simulink model "satellite_adcs_model"  (R2014b)
settings: Solver=ode3  StartTime=0.0  StopTime=tdur  FixedStep=dt  RelTol=1e-3
values from neighbouring files (symbols this model uses):
  CTRL_DT_MODE = 3    [satellite_adcs_run.m]
  CTRL_PT1_MODE = 5    [satellite_adcs_run.m]
  CTRL_PT2_MODE = 5    [satellite_adcs_run.m]
  CTRL_SWITCH1 = 1    [satellite_adcs_run.m]
  CTRL_SWITCH2 = P/2    [satellite_adcs_run.m]
  dt = CONST.dt    [extended_kalman_filter.m]    (also in filter_kalman_extended.m; filter_kalman_sequential.m; filter_kalman_unscented.m; satellite_adcs_run.m = 1)
  dt_gyro = 0.1    [satellite_adcs_run.m]
  dt_mg = dt    (= 1)    [satellite_adcs_run.m]
  dt_ss = dt    (= 1)    [satellite_adcs_run.m]
  dt_st = dt    (= 1)    [satellite_adcs_run.m]
  dt_ts = dt    (= 1)    [satellite_adcs_run.m]
  GYRO_Bias = [0.5;0.2;-0.3]*pi/180    [satellite_adcs_run.m]
  q_B_I_0 = qinvert(q_I_B_0,'xyzw')    [satellite_adcs_run.m]
  R_G_B = dcm(2,pi/2)    [satellite_adcs_run.m]
  R_S1_B = dcm(SSaxis(1),SSangles(1))    [satellite_adcs_run.m]
  R_S2_B = dcm(SSaxis(2),SSangles(2))    [satellite_adcs_run.m]
  R_S3_B = dcm(SSaxis(3),SSangles(3))    [satellite_adcs_run.m]
  R_S4_B = dcm(SSaxis(4),SSangles(4))    [satellite_adcs_run.m]
  sigMag = 1.25e-7    (= 1.25e-07)    [satellite_adcs_run.m]
  sigSS = 0.01*pi/180    (= 0.000174532925199)    [satellite_adcs_run.m]
  Taero_toggle = 0    [satellite_adcs_run.m]
  Tcontrol_toggle = 1    [satellite_adcs_run.m]
  temp_coeff = [0.01; 0.02; 0.005]*pi/180    [satellite_adcs_run.m]
  temp_ref = 20    [satellite_adcs_run.m]
  Tgg_toggle = 0    [satellite_adcs_run.m]
  Tsolar_toggle = 0    [satellite_adcs_run.m]
  Ug = dcm(3,GYRO_Mis(3))*dcm(2,GYRO_Mis(2))*dcm(1,GYRO_Mis(1))    [satellite_adcs_run.m]
  Umg = eye(3) + Gmg    [satellite_adcs_run.m]    (also in sensor_mag.m = CONST.Umg)
  update_st1 = 2    [satellite_adcs_run.m]
  update_st2 = 2    [satellite_adcs_run.m]
  Var_ARW = N_ARW^2    (= 2.56183250041e-09)    [satellite_adcs_run.m]
  Var_RRW = K_RRW^2/3    (= 4.06156559716e-12)    [satellite_adcs_run.m]
  varTemp = sigTemp^2    (= 4e-06)    [satellite_adcs_run.m]
  VarW = N_W^2    (= 3.04617419787e-22)    [satellite_adcs_run.m]
  w_B_BI_0 = w_B_BO_0 + w_B_OI_0    [satellite_adcs_run.m]
  wdot_B_BI_tgt = [0;0;0]    [satellite_adcs_run.m]
undefined symbols (not defined in the file or in its folder): magnitude, R_0, V_0, varST_x, varST_y, varST_z
libraries: simulink x6
(part 1 of 2)
settings Model: Creator=Goh  LastModifiedBy=root
settings DataIOCC: LimitDataPoints=off  SaveTime=off
settings OptimizationCC: BlockReduction=off  BooleanDataType=off  UseDivisionForNetSlopeComputation=off  SimCompilerOptimization=off
settings DebuggingCC: SaveWithParameterizedLinksMsg=none  UnderspecifiedInitializationDetection=Classic  MergeDetectMultiDrivingBlocksExec=none  SignalResolutionControl=TryResolveAllWithWarning  SolverPrmCheckMsg=none  FcnCallInpInsideContextMsg=error  FrameProcessingCompatibilityMsg=error  SFExecutionAtInitializationDiag=none
settings HardwareCC: ProdBitPerSizeT=32  ProdBitPerPtrDiffT=32  TargetUnknown=on
settings RTWCC: RTWCompilerOptimization=off
settings CodeAppCC: StateflowObjectComments=on
settings ConfigComp: CovMetricSettings=dw  CovHtmlReporting=on  CovSaveCumulativeToWorkspaceVar=on  CovSaveSingleToWorkspaceVar=on  CovExternalEMLEnable=off  CovSFcnEnable=off

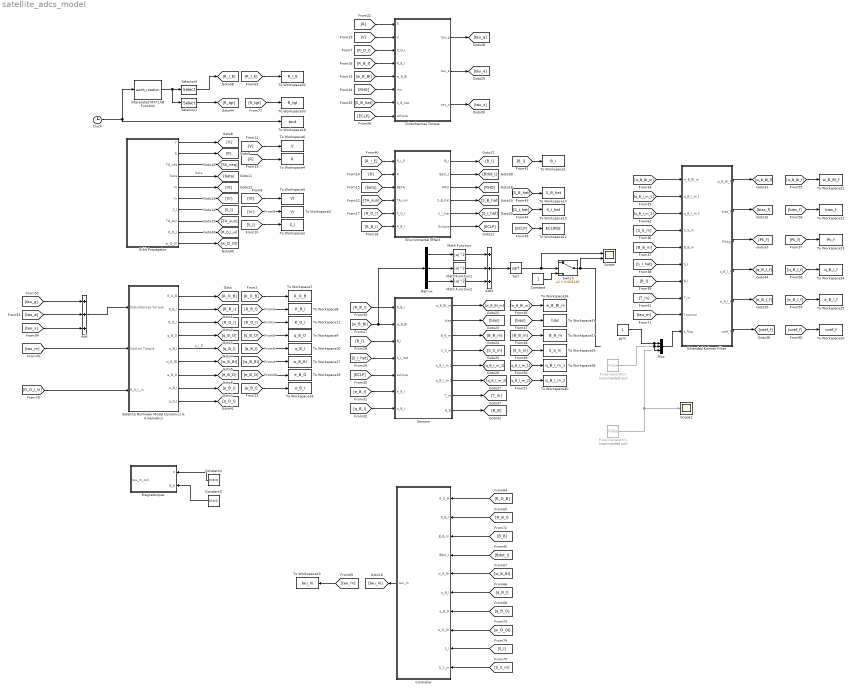
== system satellite_adcs_model ==
  Add : Sum  Inputs=+++
  Add1 : Sum  Inputs=3
  Clock : Clock
  Constant : Constant
  Constant3 : Constant  Value=[0;0;0]
  Constant4 : Constant  Value=[0;0;0]
  Controller : Subsystem
  Demux : Demux  Outputs=3
  Disturbances Torque : Subsystem
  Environmental Effect : Subsystem
  Extended Kalman Filter : Subsystem
  Interpreted MATLAB Function : MATLABFcn  MATLABFcn=earth_rotation  OutputDimensions=[3,4]  Output1D=off
  Magnetorquer : Subsystem
  Math Function : Math  Operator=magnitude^2  SaturateOnIntegerOverflow=on
  Math Function1 : Math  Operator=magnitude^2  SaturateOnIntegerOverflow=on
  Math Function2 : Math  Operator=magnitude^2  SaturateOnIntegerOverflow=on
  Mux : Mux  Inputs=3
  Orbit Propagator : Subsystem
  Pulse Generator : DiscretePulseGenerator  Commented=on  PulseType=Time based  Period=update_st1  PulseWidth=dt/update_st1*100
  Pulse Generator1 : DiscretePulseGenerator  Commented=on  PulseType=Time based  Period=update_st2  PulseWidth=dt/update_st2*100
  Satellite Nonlinear Model Dynamics & Kinematics : Subsystem
  Scope : Scope  NumInputPorts=2
  Scope1 : Scope
  Selector1 : Selector  NumberOfDimensions=2  InputPortWidth=9  IndexOptions=Index vector (dialog),Index vector (dialog)  Indices=1:3,4  OutputSizes=1,1
  Selector5 : Selector  NumberOfDimensions=2  InputPortWidth=9  IndexOptions=Index vector (dialog),Index vector (dialog)  Indices=1:3,1:3  OutputSizes=1,1
  Sensors : Subsystem
  Sqrt : Sqrt  SaturateOnIntegerOverflow=on
  Switch : Switch  Criteria=u2 > Threshold  Threshold=0.005236
  To Workspace1 : ToWorkspace  VariableName=B_I  SampleTime=dt
  To Workspace10 : ToWorkspace  VariableName=q_B_I  SampleTime=dt
  To Workspace11 : ToWorkspace  VariableName=R_O_I  SampleTime=dt
  To Workspace12 : ToWorkspace  VariableName=ECLIPSE  SampleTime=dt
      settings: Save2DSignal=2-D array (concatenate along first dimension)
  To Workspace13 : ToWorkspace  VariableName=S_I_hat  SampleTime=dt
  To Workspace14 : ToWorkspace  VariableName=S_B_hat  SampleTime=dt
  To Workspace15 : ToWorkspace  VariableName=tau_m  SampleTime=-1
  To Workspace16 : ToWorkspace  VariableName=tout  SampleTime=dt
  To Workspace17 : ToWorkspace  VariableName=w_B_BI  SampleTime=dt
  To Workspace18 : ToWorkspace  VariableName=e_B_I  SampleTime=dt
  To Workspace19 : ToWorkspace  VariableName=e_B_O  SampleTime=dt
  To Workspace2 : ToWorkspace  VariableName=S_I  SampleTime=dt
  To Workspace20 : ToWorkspace  VariableName=coef_f  SampleTime=dt
  To Workspace21 : ToWorkspace  VariableName=w_B_BI_f  SampleTime=dt
  To Workspace22 : ToWorkspace  VariableName=bias_f  SampleTime=dt
  To Workspace23 : ToWorkspace  VariableName=Pk_f  SampleTime=dt
  To Workspace24 : ToWorkspace  VariableName=q_B_I_f  SampleTime=dt
  To Workspace25 : ToWorkspace  VariableName=e_B_I_f  SampleTime=dt
  To Workspace26 : ToWorkspace  VariableName=w_B_BI_m  SampleTime=dt
  To Workspace27 : ToWorkspace  VariableName=B_B_m  SampleTime=dt
  To Workspace28 : ToWorkspace  VariableName=q_B_I_m_1  SampleTime=dt
  To Workspace29 : ToWorkspace  VariableName=S_S_m  SampleTime=dt
  To Workspace3 : ToWorkspace  VariableName=Vr  SampleTime=dt
  To Workspace30 : ToWorkspace  VariableName=q_B_I_m_2  SampleTime=dt
  To Workspace31 : ToWorkspace  VariableName=bias  SampleTime=dt
  To Workspace32 : ToWorkspace  VariableName=R_I_E  SampleTime=dt
  To Workspace33 : ToWorkspace  VariableName=R_tgt  SampleTime=dt
  To Workspace4 : ToWorkspace  VariableName=R  SampleTime=dt
  To Workspace5 : ToWorkspace  VariableName=Vt  SampleTime=dt
  To Workspace6 : ToWorkspace  VariableName=V  SampleTime=dt
  To Workspace7 : ToWorkspace  VariableName=R_O_B  SampleTime=dt
  To Workspace8 : ToWorkspace  VariableName=R_B_I  SampleTime=dt
  To Workspace9 : ToWorkspace  VariableName=q_B_O  SampleTime=dt
  "gyro " : Constant
  wires:
  Satellite Nonlinear Model Dynamics & Kinematics/1(R_O_B) -> [R_O_B]
  Satellite Nonlinear Model Dynamics & Kinematics/2(R_B_I) -> [R_B_I]
  Satellite Nonlinear Model Dynamics & Kinematics/4(q_B_O) -> [q_B_O]
  Satellite Nonlinear Model Dynamics & Kinematics/5(q_B_I) -> [q_B_I]  "q_I_B"
  Satellite Nonlinear Model Dynamics & Kinematics/6(w_B_BI) -> [w_B_BI]
  Satellite Nonlinear Model Dynamics & Kinematics/7(e_B_O) -> [e_B_O]
  Satellite Nonlinear Model Dynamics & Kinematics/8(e_B_I) -> [e_B_I]
  Orbit Propagator/7("S_I ") -> [S_I]
  Orbit Propagator/8(TA_sun) -> [TA_sun]
  Orbit Propagator/1(V) -> [V]
  Orbit Propagator/2(R) -> [R]
  Orbit Propagator/3(TA_veq) -> [TA_veq]
  Orbit Propagator/4(beta) -> [beta]  "beta"
  Orbit Propagator/5(Vt) -> [Vt]
  Orbit Propagator/6(Vr) -> [Vr]
  Environmental Effect/1(B_I) -> [B_I]
  Environmental Effect/3(RHO) -> [RHO]
  Environmental Effect/4(S_B_hat) -> [S_B_hat]
  Environmental Effect/5(S_I_hat) -> [S_I_hat]
  Environmental Effect/6(Eclipse) -> [ECLP]
  Sensors/3(B_B_m) -> [B_B_m]
  Sensors/2(bias) -> [bias]
  Sensors/1(w_B_BI_m) -> [w_B_BI_m]
  Sensors/4(S_S_m) -> [S_S_m]
  Sensors/5(q_B_I_m 1) -> [q_B_I_m_1]
  Disturbances Torque/1(tau_g) -> [tau_g]
  Disturbances Torque/2(tau_a) -> [tau_a]
  Disturbances Torque/3(tau_s) -> [tau_s]
  Extended Kalman Filter/1(w_B_BI_f) -> [w_B_BI_f]
  Extended Kalman Filter/2(bias_f) -> [bias_f]
  Extended Kalman Filter/3(Pdiag) -> [Pk_f]
  Extended Kalman Filter/4(q_B_I_f) -> [q_B_I_f]
  Extended Kalman Filter/5(e_B_I_f) -> [e_B_I_f]
  [R_O_B] -> To Workspace7/1
  [R_B_I] -> To Workspace8/1
  [R_O_I] -> To Workspace11/1
  [q_B_O] -> To Workspace9/1
  [q_B_I] -> To Workspace10/1
  [w_B_BI] -> To Workspace17/1
  [e_B_O] -> To Workspace19/1
  [e_B_I] -> To Workspace18/1
  [Vt] -> To Workspace5/1
  [Vr] -> To Workspace3/1
  [S_I] -> To Workspace2/1
  [R] -> To Workspace4/1
  [V] -> To Workspace6/1
  [beta] -> Environmental Effect/3(BETA)
  [TA_sun] -> Environmental Effect/4(TA_sun)
  [R] -> Environmental Effect/2(R)
  [R_O_I] -> Environmental Effect/5(R_O_I)
  [R_B_I] -> Environmental Effect/6(R_B_I)
  [RHO] -> Disturbances Torque/6(rho)
  [w_B_BI] -> Disturbances Torque/5(w_B_BI)
  [R_B_I] -> Disturbances Torque/4(R_B_I)
  [R_O_I] -> Disturbances Torque/3(R_O_I)
  [V] -> Disturbances Torque/2(V)
  [R] -> Disturbances Torque/1(R)
  [S_B_hat] -> Disturbances Torque/7(S_B_hat)
  [ECLP] -> Disturbances Torque/8(eclipse)
  [R_B_I] -> Sensors/1(R_B_I)
  [w_B_BI] -> Demux/1, Sensors/2(w_B_BI)
  [B_I] -> Sensors/3(B_I)
  [e_B_I] -> Sensors/6(e_B_I)
  [q_B_I] -> Sensors/7(q_B_I)
  [S_I_hat] -> Sensors/4(S_I_hat)
  [ECLP] -> Sensors/5(eclipse)
  [B_B_m] -> Extended Kalman Filter/5(B_B_m)
  [S_I_hat] -> Extended Kalman Filter/6(S_I)
  [B_I] -> Extended Kalman Filter/7(B_I)
  [S_S_m] -> Extended Kalman Filter/4(S_S_m)
  [w_B_BI_m] -> Extended Kalman Filter/1(w_B_BI_m)
  [q_B_I_m_1] -> Extended Kalman Filter/2(q_B_I_m 1)
  [B_I] -> To Workspace1/1
  [S_B_hat] -> To Workspace14/1
  [S_I_hat] -> To Workspace13/1
  [ECLP] -> To Workspace12/1
  [w_B_BI_m] -> To Workspace26/1
  [q_B_I_m_1] -> To Workspace28/1
  [bias] -> To Workspace31/1
  [S_S_m] -> To Workspace29/1
  [B_B_m] -> To Workspace27/1
  [tau_s] -> Add/3
  [tau_g] -> Add/1
  [w_B_BI_f] -> To Workspace21/1
  [bias_f] -> To Workspace22/1
  [Pk_f] -> To Workspace23/1
  [q_B_I_f] -> To Workspace24/1
  [e_B_I_f] -> To Workspace25/1
  [coef_f] -> To Workspace20/1
  Extended Kalman Filter/6(coef_f) -> [coef_f]
  Sensors/7(T_m) -> [T_m]
  [T_m] -> Extended Kalman Filter/8(T_m)
  [q_B_I_m_2] -> To Workspace30/1
  Sensors/6(q_B_I_m 2) -> [q_B_I_m_2]
  [q_B_I_m_2] -> Extended Kalman Filter/3(q_B_I_m 2)
  [tau_a] -> Add/2
  [R_I_E] -> To Workspace32/1
  [R_I_E] -> Environmental Effect/1(R_I_E)
  Mux/1 -> Extended Kalman Filter/10(s_flag)
  [w_B_BI] -> Controller/5(w_B_BI)
  [tau_m] -> To Workspace15/1
  Controller/1(tau_m) -> [tau_m]
  [R_O_B] -> Controller/1(R_O_B)
  [B_B] -> Controller/3(B_B_m)
  [R_B_I] -> Controller/2(R_B_I)
  [tau_m] -> Extended Kalman Filter/9(Tcontrol)
  Environmental Effect/2(Bdot_I) -> [Bdot_I]
  [Bdot_I] -> Controller/4(Bdot_I)
  "gyro "/1 -> Mux/3, Mux/2, Mux/1
  Pulse Generator1/1 -> Scope1/1
  Switch/1 -> Scope/2
  Demux/1 -> Math Function/1
  Demux/2 -> Math Function1/1
  Demux/3 -> Math Function2/1
  Math Function/1 -> Add1/1
  Math Function1/1 -> Add1/2
  Math Function2/1 -> Add1/3
  Add1/1 -> Sqrt/1
  Sqrt/1 -> Switch/2, Scope/1
  Constant/1 -> Switch/3
  Clock/1 -> To Workspace16/1, Interpreted MATLAB Function/1
  [q_B_I] -> Controller/6(q_B_I)
  [q_B_O] -> Controller/7(q_B_O)
  Satellite Nonlinear Model Dynamics & Kinematics/9(q_O_I) -> [q_O_I]
  Satellite Nonlinear Model Dynamics & Kinematics/3(R_O_I) -> [R_O_I]
  Orbit Propagator/10(w_O_OI) -> [w_O_OI]
  [w_O_OI] -> Controller/8(w_O_OI)
  [S_I] -> Controller/9(S_I)
  [S_S_m] -> Controller/10(S_S_m)
  Pulse Generator/1 -> ?
  Constant4/1 -> Magnetorquer/1(V)
  Constant3/1 -> Magnetorquer/2(B_b)
  Sensors/8(B_B) -> [B_B]
  Orbit Propagator/9(R_O_I) -> [R_O_I_in]
  [R_O_I_in] -> Satellite Nonlinear Model Dynamics & Kinematics/3(R_O_I_in)
  Add/1 -> Satellite Nonlinear Model Dynamics & Kinematics/1(Disturbances Torque)
  Interpreted MATLAB Function/1 -> Selector1/1, Selector5/1
  [tau_m] -> Satellite Nonlinear Model Dynamics & Kinematics/2(Control Torque)
  [R_tgt] -> To Workspace33/1
  Selector5/1 -> [R_I_E]
  Selector1/1 -> [R_tgt]

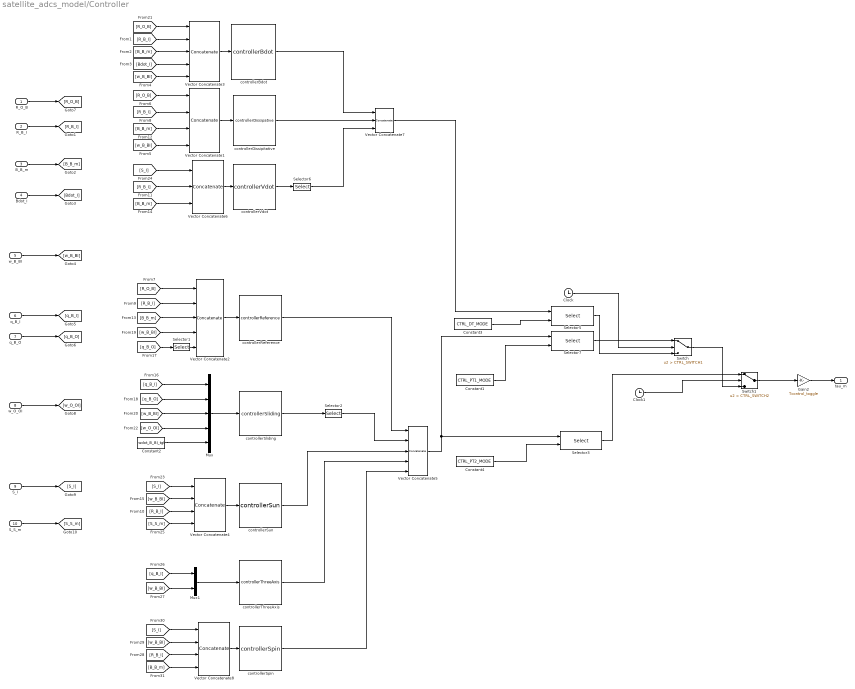
== system satellite_adcs_model/Controller ==
  R_O_B : Inport
  R_B_I : Inport  Port=2
  B_B_m : Inport  Port=3
  Bdot_I : Inport  Port=4
  w_B_BI : Inport  Port=5
  q_B_I : Inport  Port=6
  q_B_O : Inport  Port=7
  w_O_OI : Inport  Port=8
  S_I : Inport  Port=9
  S_S_m : Inport  Port=10
  Clock : Clock
  Clock1 : Clock
  Constant1 : Constant  Value=CTRL_PT1_MODE  VectorParams1D=off
  Constant2 : Constant  Value=wdot_B_BI_tgt  VectorParams1D=off
  Constant3 : Constant  Value=CTRL_DT_MODE  VectorParams1D=off
  Constant4 : Constant  Value=CTRL_PT2_MODE  VectorParams1D=off
  Gain2 : Gain  Gain=Tcontrol_toggle
  Mux : Mux  Inputs=5
  Mux1 : Mux  Inputs=2
  Selector1 : Selector  NumberOfDimensions=2  InputPortWidth=3  IndexOptions=Index vector (dialog),Index vector (dialog)  Indices=[1:3],1  OutputSizes=1,1
  Selector2 : Selector  NumberOfDimensions=2  InputPortWidth=3  IndexOptions=Index vector (dialog),Index vector (dialog)  Indices=[1:3],1  OutputSizes=1,1
  Selector3 : Selector  NumberOfDimensions=2  InputPortWidth=3  IndexOptions=Select all,Index vector (port)  Indices=[1 3],1  OutputSizes=1,1
  Selector5 : Selector  NumberOfDimensions=2  InputPortWidth=3  IndexOptions=Select all,Index vector (port)  Indices=[1 3],1  OutputSizes=1,1
  Selector6 : Selector  NumberOfDimensions=2  InputPortWidth=3  IndexOptions=Index vector (dialog),Index vector (dialog)  Indices=[1:3],1  OutputSizes=1,1
  Selector7 : Selector  NumberOfDimensions=2  InputPortWidth=3  IndexOptions=Select all,Index vector (port)  Indices=[1 3],1  OutputSizes=1,1
  Switch : Switch  Criteria=u2 > Threshold  Threshold=CTRL_SWITCH1
  Switch1 : Switch  Criteria=u2 > Threshold  Threshold=CTRL_SWITCH2
  Vector Concatenate1 : Concatenate  NumInputs=4  Mode=Multidimensional array  ConcatenateDimension=2
  Vector Concatenate2 : Concatenate  NumInputs=5  Mode=Multidimensional array  ConcatenateDimension=2
  Vector Concatenate3 : Concatenate  NumInputs=5  Mode=Multidimensional array  ConcatenateDimension=2
  Vector Concatenate4 : Concatenate  NumInputs=4  Mode=Multidimensional array  ConcatenateDimension=2
  Vector Concatenate5 : Concatenate  NumInputs=5  Mode=Multidimensional array  ConcatenateDimension=2
  Vector Concatenate6 : Concatenate  NumInputs=3  Mode=Multidimensional array  ConcatenateDimension=2
  Vector Concatenate7 : Concatenate  NumInputs=3  Mode=Multidimensional array  ConcatenateDimension=2
  Vector Concatenate8 : Concatenate  NumInputs=4  Mode=Multidimensional array  ConcatenateDimension=2
  controllerBdot : MATLABFcn  MATLABFcn=controllerBdot  OutputDimensions=[3,1]  Output1D=off
  controllerDissipitative : MATLABFcn  MATLABFcn=controllerDissipative  OutputDimensions=[3,1]  Output1D=off
  controllerReference : MATLABFcn  MATLABFcn=controllerReference  OutputDimensions=[3,1]  Output1D=off
  "controllerSliding " : MATLABFcn  MATLABFcn=controllerSliding  OutputDimensions=[3,3]  Output1D=off
  controllerSpin : MATLABFcn  MATLABFcn=controllerSpin  OutputDimensions=[3,1]  Output1D=off
  controllerSun : MATLABFcn  MATLABFcn=controllerSun  OutputDimensions=[3,1]  Output1D=off
  controllerThreeAxis : MATLABFcn  MATLABFcn=controllerThreeAxis  OutputDimensions=[3,1]  Output1D=off
  controllerVdot : MATLABFcn  MATLABFcn=controllerVdot  OutputDimensions=[6,1]  Output1D=off
  tau_m : Outport
  wires:
  Vector Concatenate1/1 -> controllerDissipitative/1
  R_O_B/1 -> [R_O_B]
  R_B_I/1 -> [R_B_I]
  B_B_m/1 -> [B_B_m]
  w_B_BI/1 -> [w_B_BI]
  Vector Concatenate2/1 -> controllerReference/1
  controllerReference/1 -> Vector Concatenate5/1
  Clock/1 -> Switch/2
  Switch/1 -> Switch1/3
  Vector Concatenate3/1 -> controllerBdot/1
  controllerBdot/1 -> Vector Concatenate7/1
  controllerDissipitative/1 -> Vector Concatenate7/2
  Vector Concatenate7/1 -> Selector5/1
  Mux/1 -> "controllerSliding "/1
  Constant2/1 -> Mux/5
  Selector7/1 -> Switch/1
  Vector Concatenate4/1 -> controllerSun/1
  Vector Concatenate5/1 -> Selector3/1, Selector7/1
  Selector1/1 -> Vector Concatenate2/5
  "controllerSliding "/1 -> Selector2/1
  Selector2/1 -> Vector Concatenate5/2
  controllerSun/1 -> Vector Concatenate5/3
  Constant1/1 -> Selector7/2
  Vector Concatenate6/1 -> controllerVdot/1
  controllerVdot/1 -> Selector6/1
  Selector5/1 -> Switch/3
  Constant3/1 -> Selector5/2
  Selector6/1 -> Vector Concatenate7/3
  [R_O_B] -> Vector Concatenate3/1
  [R_B_I] -> Vector Concatenate3/2
  [B_B_m] -> Vector Concatenate3/3
  [Bdot_I] -> Vector Concatenate3/4
  Bdot_I/1 -> [Bdot_I]
  [w_B_BI] -> Vector Concatenate3/5
  [w_B_BI] -> Vector Concatenate1/4
  [R_O_B] -> Vector Concatenate1/1
  [R_O_B] -> Vector Concatenate2/1
  [R_B_I] -> Vector Concatenate1/2
  [R_B_I] -> Vector Concatenate2/2
  [R_B_I] -> Vector Concatenate4/3
  [R_B_I] -> Vector Concatenate6/2
  [B_B_m] -> Vector Concatenate1/3
  [B_B_m] -> Vector Concatenate2/3
  [B_B_m] -> Vector Concatenate6/3
  [w_B_BI] -> Vector Concatenate4/2
  q_B_I/1 -> [q_B_I]
  [q_B_I] -> Mux/1
  q_B_O/1 -> [q_B_O]
  [q_B_O] -> Selector1/1
  [q_B_O] -> Mux/2
  [w_B_BI] -> Vector Concatenate2/4
  [w_B_BI] -> Mux/3
  w_O_OI/1 -> [w_O_OI]
  [w_O_OI] -> Mux/4
  S_I/1 -> [S_I]
  [S_I] -> Vector Concatenate4/1
  [S_I] -> Vector Concatenate6/1
  S_S_m/1 -> [S_S_m]
  [S_S_m] -> Vector Concatenate4/4
  controllerThreeAxis/1 -> Vector Concatenate5/4
  Mux1/1 -> controllerThreeAxis/1
  [q_B_I] -> Mux1/1
  [w_B_BI] -> Mux1/2
  Clock1/1 -> Switch1/2
  Switch1/1 -> Gain2/1
  Selector3/1 -> Switch1/1
  Constant4/1 -> Selector3/2
  Gain2/1 -> tau_m/1
  Vector Concatenate8/1 -> controllerSpin/1
  [w_B_BI] -> Vector Concatenate8/2
  [S_I] -> Vector Concatenate8/1
  [R_B_I] -> Vector Concatenate8/3
  [B_B_m] -> Vector Concatenate8/4
  controllerSpin/1 -> Vector Concatenate5/5

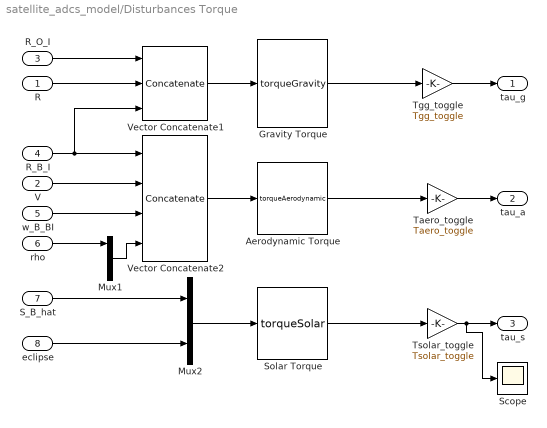
== system satellite_adcs_model/Disturbances Torque ==
  R : Inport
  V : Inport  Port=2
  R_O_I : Inport  Port=3
  R_B_I : Inport  Port=4
  w_B_BI : Inport  Port=5
  rho : Inport  Port=6
  S_B_hat : Inport  Port=7
  eclipse : Inport  Port=8
  Aerodynamic Torque : MATLABFcn  MATLABFcn=torqueAerodynamic  OutputDimensions=[3,1]  Output1D=off
  Gravity Torque : MATLABFcn  MATLABFcn=torqueGravity  OutputDimensions=[3,1]  Output1D=off
  Mux1 : Mux  Inputs=3
  Mux2 : Mux  Inputs=2
  Scope : Scope
      settings: YMin=-0.0000000000000000000000009  YMax=0.0000000000000000000000012  SaveName=ScopeData8
  Solar Torque : MATLABFcn  MATLABFcn=torqueSolar  OutputDimensions=[3,1]  Output1D=off
  Taero_toggle : Gain  Gain=Taero_toggle
  Tgg_toggle : Gain  Gain=Tgg_toggle
  Tsolar_toggle : Gain  Gain=Tsolar_toggle
  Vector Concatenate1 : Concatenate  NumInputs=3  Mode=Multidimensional array  ConcatenateDimension=2
  Vector Concatenate2 : Concatenate  NumInputs=4  Mode=Multidimensional array  ConcatenateDimension=2
  tau_g : Outport
  tau_a : Outport  Port=2
  tau_s : Outport  Port=3
  wires:
  Vector Concatenate2/1 -> Aerodynamic Torque/1
  Mux1/1 -> Vector Concatenate2/4
  Solar Torque/1 -> Tsolar_toggle/1
  Vector Concatenate1/1 -> Gravity Torque/1
  Mux2/1 -> Solar Torque/1
  S_B_hat/1 -> Mux2/1
  w_B_BI/1 -> Vector Concatenate2/3
  R_B_I/1 -> Vector Concatenate1/3, Vector Concatenate2/1
  V/1 -> Vector Concatenate2/2
  R/1 -> Vector Concatenate1/2
  R_O_I/1 -> Vector Concatenate1/1
  rho/1 -> Mux1/1
  Aerodynamic Torque/1 -> Taero_toggle/1
  eclipse/1 -> Mux2/2
  Tgg_toggle/1 -> tau_g/1
  Taero_toggle/1 -> tau_a/1
  Tsolar_toggle/1 -> Scope/1, tau_s/1
  Gravity Torque/1 -> Tgg_toggle/1

== system satellite_adcs_model/Environmental Effect ==
  R_I_E : Inport
  R : Inport  Port=2
  BETA : Inport  Port=3
  TA_sun : Inport  Port=4
  R_O_I : Inport  Port=5
  R_B_I : Inport  Port=6
  DENSITY : Subsystem
  MAGNETIC FIELD : Subsystem
  SUN : Subsystem
  B_I : Outport
  Bdot_I : Outport  Port=2
  RHO : Outport  Port=3
  S_B_hat : Outport  Port=4
  S_I_hat : Outport  Port=5
  Eclipse : Outport  Port=6
  wires:
  R/1 -> MAGNETIC FIELD/2(R), SUN/1(R), DENSITY/1(R)
  TA_sun/1 -> SUN/2(S_TA), DENSITY/2(S_TA)
  BETA/1 -> SUN/3(BETA), DENSITY/3(BETA)
  R_O_I/1 -> SUN/4(R_O_I)
  R_B_I/1 -> SUN/5(R_B_I)
  SUN/1(S_B_hat) -> S_B_hat/1
  SUN/2(S_I_hat) -> S_I_hat/1
  SUN/3(Eclipse) -> Eclipse/1
  DENSITY/1(RHO) -> RHO/1
  R_I_E/1 -> MAGNETIC FIELD/1(R_I_E)
  MAGNETIC FIELD/1(B_I) -> B_I/1
  MAGNETIC FIELD/2(Bdot_I) -> Bdot_I/1

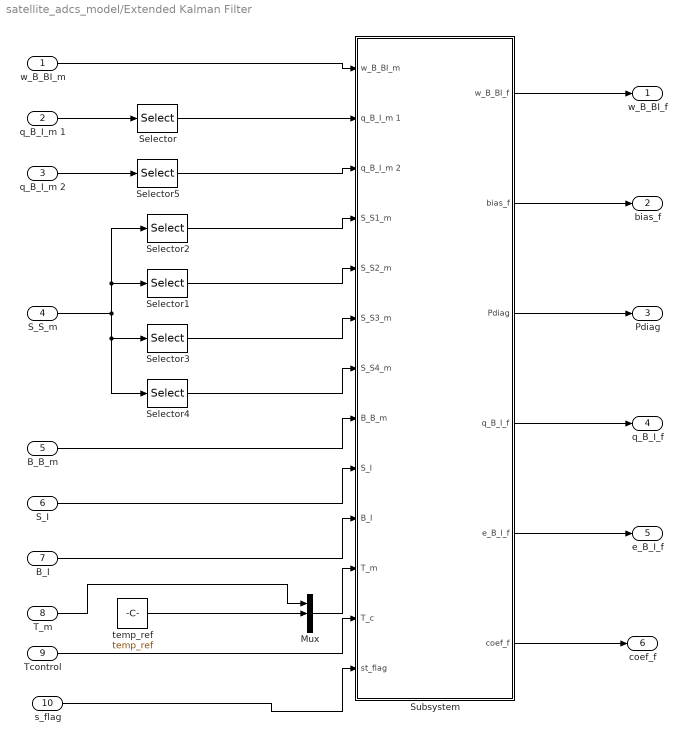
== system satellite_adcs_model/Extended Kalman Filter ==
  w_B_BI_m : Inport
  q_B_I_m 1 : Inport  Port=2
  q_B_I_m 2 : Inport  Port=3
  S_S_m : Inport  Port=4
  B_B_m : Inport  Port=5
  S_I : Inport  Port=6
  B_I : Inport  Port=7
  T_m : Inport  Port=8
  Tcontrol : Inport  Port=9
  s_flag : Inport  Port=10
  Mux : Mux  Inputs=3
  Selector : Selector  InputPortWidth=4  Indices=[1:3]
  Selector1 : Selector  NumberOfDimensions=2  InputPortWidth=4  IndexOptions=Index vector (dialog),Index vector (dialog)  Indices=[1:3],2  OutputSizes=1,1
  Selector2 : Selector  NumberOfDimensions=2  InputPortWidth=4  IndexOptions=Index vector (dialog),Index vector (dialog)  Indices=[1:3],1  OutputSizes=1,1
  Selector3 : Selector  NumberOfDimensions=2  InputPortWidth=4  IndexOptions=Index vector (dialog),Index vector (dialog)  Indices=[1:3],3  OutputSizes=1,1
  Selector4 : Selector  NumberOfDimensions=2  InputPortWidth=4  IndexOptions=Index vector (dialog),Index vector (dialog)  Indices=[1:3],4  OutputSizes=1,1
  Selector5 : Selector  InputPortWidth=4  Indices=[1:3]
  Subsystem : Subsystem
  temp_ref : Constant  Value=temp_ref
  w_B_BI_f : Outport
  bias_f : Outport  Port=2
  Pdiag : Outport  Port=3
  q_B_I_f : Outport  Port=4
  e_B_I_f : Outport  Port=5
  coef_f : Outport  Port=6
  wires:
  q_B_I_m 1/1 -> Selector/1
  w_B_BI_m/1 -> Subsystem/1(w_B_BI_m)
  Selector2/1 -> Subsystem/4(S_S1_m)
  Selector1/1 -> Subsystem/5(S_S2_m)
  B_B_m/1 -> Subsystem/8(B_B_m)
  B_I/1 -> Subsystem/10(B_I)
  S_I/1 -> Subsystem/9(S_I)
  Subsystem/1(w_B_BI_f) -> w_B_BI_f/1
  Subsystem/2(bias_f) -> bias_f/1
  Subsystem/3(Pdiag) -> Pdiag/1
  Subsystem/4(q_B_I_f) -> q_B_I_f/1
  Subsystem/5(e_B_I_f) -> e_B_I_f/1
  S_S_m/1 -> Selector4/1, Selector3/1, Selector2/1, Selector1/1
  Selector3/1 -> Subsystem/6(S_S3_m)
  Selector4/1 -> Subsystem/7(S_S4_m)
  Subsystem/6(coef_f) -> coef_f/1
  T_m/1 -> Mux/1
  Mux/1 -> Subsystem/11(T_m)
  temp_ref/1 -> Mux/2
  q_B_I_m 2/1 -> Selector5/1
  Selector5/1 -> Subsystem/3(q_B_I_m 2)
  Tcontrol/1 -> Subsystem/12(T_c)
  Selector/1 -> Subsystem/2(q_B_I_m 1)
  s_flag/1 -> Subsystem/13(st_flag)

== system satellite_adcs_model/Magnetorquer ==
  V : Inport
  B_b : Inport  Port=2
  Magnetorquer : MATLABFcn  MATLABFcn=actuatorMagnetorquer  OutputDimensions=[3,1]  Output1D=off
  Mux : Mux  Inputs=2
  tau_m_coil : Outport
  wires:
  V/1 -> Mux/1
  Mux/1 -> Magnetorquer/1
  Magnetorquer/1 -> tau_m_coil/1
  B_b/1 -> Mux/2

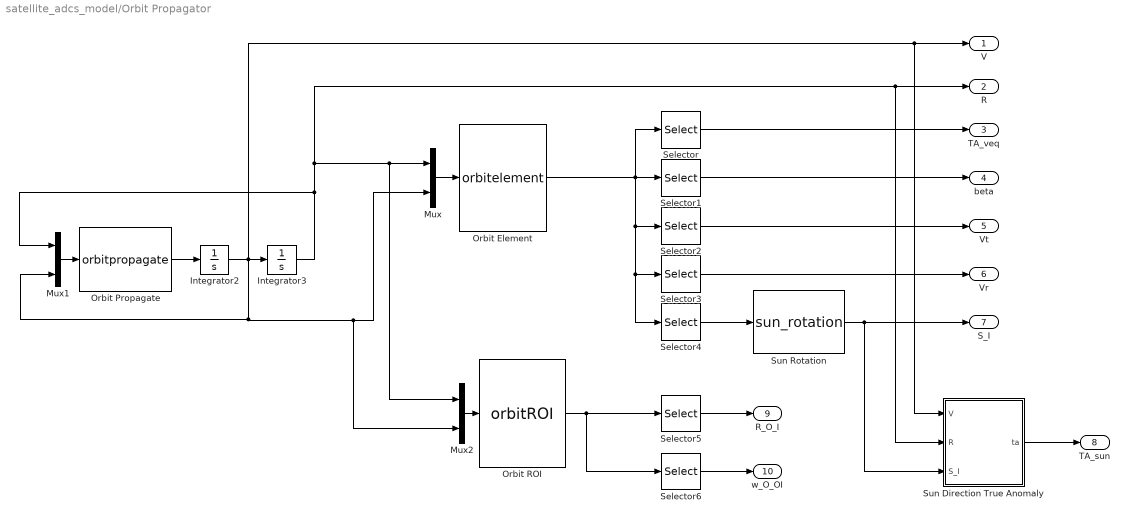
== system satellite_adcs_model/Orbit Propagator ==
  Integrator2 : Integrator  InitialCondition=V_0
  Integrator3 : Integrator  InitialCondition=R_0
  Mux : Mux  Inputs=2
  Mux1 : Mux  Inputs=2
  Mux2 : Mux  Inputs=2
  Orbit Element : MATLABFcn  MATLABFcn=orbitelement  Output1D=off
  Orbit Propagate : MATLABFcn  MATLABFcn=orbitpropagate  OutputDimensions=[3,1]  Output1D=off
  Orbit ROI : MATLABFcn  MATLABFcn=orbitROI  OutputDimensions=[3,4]  Output1D=off
  Selector : Selector  InputPortWidth=9
  Selector1 : Selector  InputPortWidth=9  Indices=2
  Selector2 : Selector  InputPortWidth=9  Indices=[3:5]
  Selector3 : Selector  InputPortWidth=9  Indices=[6:8]
  Selector4 : Selector  InputPortWidth=9  Indices=9
  Selector5 : Selector  NumberOfDimensions=2  InputPortWidth=9  IndexOptions=Index vector (dialog),Index vector (dialog)  Indices=1:3,1:3  OutputSizes=1,1
  Selector6 : Selector  NumberOfDimensions=2  InputPortWidth=9  IndexOptions=Index vector (dialog),Index vector (dialog)  Indices=1:3,4  OutputSizes=1,1
  Sun Direction True Anomaly : Subsystem
  Sun Rotation : MATLABFcn  MATLABFcn=sun_rotation  OutputDimensions=[3,1]  Output1D=off
  V : Outport
  R : Outport  Port=2
  TA_veq : Outport  Port=3
  beta : Outport  Port=4
  Vt : Outport  Port=5
  Vr : Outport  Port=6
  "S_I " : Outport  Port=7
  TA_sun : Outport  Port=8
  R_O_I : Outport  Port=9
  w_O_OI : Outport  Port=10
  wires:
  Mux/1 -> Orbit Element/1
  Orbit Element/1 -> Selector/1, Selector4/1, Selector3/1, Selector2/1, Selector1/1
  Orbit Propagate/1 -> Integrator2/1
  Integrator3/1 -> Sun Direction True Anomaly/2(R), R/1, Mux2/1, Mux/1, Mux1/1
  Integrator2/1 -> Mux1/2, Mux2/2, Mux/2, Sun Direction True Anomaly/1(V), V/1, Integrator3/1
  Selector3/1 -> Vr/1
  Selector/1 -> TA_veq/1
  Selector2/1 -> Vt/1
  Selector1/1 -> beta/1
  Sun Rotation/1 -> Sun Direction True Anomaly/3(S_I), "S_I "/1
  Selector4/1 -> Sun Rotation/1
  Sun Direction True Anomaly/1(ta) -> TA_sun/1
  Mux1/1 -> Orbit Propagate/1
  Mux2/1 -> Orbit ROI/1
  Orbit ROI/1 -> Selector6/1, Selector5/1
  Selector5/1 -> R_O_I/1
  Selector6/1 -> w_O_OI/1

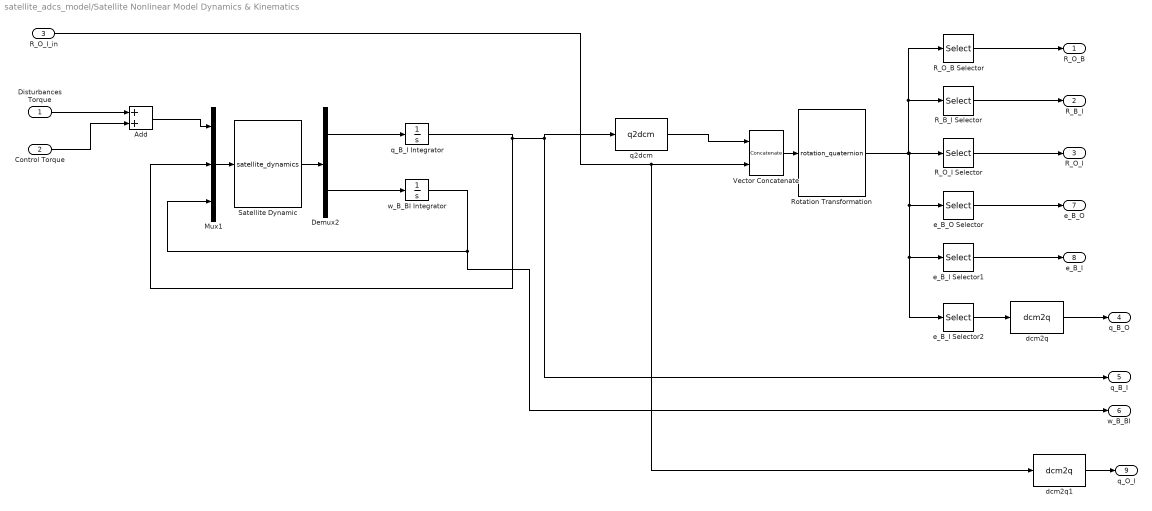
== system satellite_adcs_model/Satellite Nonlinear Model Dynamics & Kinematics ==
  Disturbances Torque : Inport
  Control Torque : Inport  Port=2
  R_O_I_in : Inport  Port=3
  " w_B_BI Integrator" : Integrator  InitialCondition=w_B_BI_0
  Add : Sum
  Demux2 : Demux  Outputs=[4 3]
  Mux1 : Mux  Inputs=[3 4 3]
  R_B_I Selector : Selector  NumberOfDimensions=2  InputPortWidth=3  IndexOptions=Index vector (dialog),Index vector (dialog)  Indices=[1:3],[4:6]  OutputSizes=1,1
  R_O_B Selector : Selector  NumberOfDimensions=2  InputPortWidth=3  IndexOptions=Index vector (dialog),Index vector (dialog)  Indices=[1:3],[1:3]  OutputSizes=1,1
  R_O_I Selector : Selector  NumberOfDimensions=2  InputPortWidth=3  IndexOptions=Index vector (dialog),Index vector (dialog)  Indices=[1:3],[7:9]  OutputSizes=1,1
  Rotation Transformation : MATLABFcn  MATLABFcn=rotation_quaternion  OutputDimensions=[3,14]  Output1D=off
  Satellite Dynamic : MATLABFcn  MATLABFcn=satellite_dynamics  OutputDimensions=[7,1]  Output1D=off
  Vector Concatenate : Concatenate  Mode=Multidimensional array  ConcatenateDimension=2
  dcm2q : MATLABFcn  MATLABFcn=dcm2q  OutputDimensions=[4,1]  Output1D=off
  dcm2q1 : MATLABFcn  MATLABFcn=dcm2q  OutputDimensions=[4,1]  Output1D=off
  e_B_I Selector1 : Selector  NumberOfDimensions=2  InputPortWidth=3  IndexOptions=Index vector (dialog),Index vector (dialog)  Indices=[1:3],11  OutputSizes=1,1
  e_B_I Selector2 : Selector  NumberOfDimensions=2  InputPortWidth=3  IndexOptions=Index vector (dialog),Index vector (dialog)  Indices=[1:3],[12:14]  OutputSizes=1,1
  e_B_O Selector : Selector  NumberOfDimensions=2  InputPortWidth=3  IndexOptions=Index vector (dialog),Index vector (dialog)  Indices=[1:3],10  OutputSizes=1,1
  q2dcm : MATLABFcn  MATLABFcn=q2dcm  OutputDimensions=[3,3]  Output1D=off
  q_B_I Integrator : Integrator  InitialCondition=q_B_I_0
  R_O_B : Outport
  R_B_I : Outport  Port=2
  R_O_I : Outport  Port=3
  q_B_O : Outport  Port=4
  q_B_I : Outport  Port=5
  w_B_BI : Outport  Port=6
  e_B_O : Outport  Port=7
  e_B_I : Outport  Port=8
  q_O_I : Outport  Port=9
  wires:
  R_O_I Selector/1 -> R_O_I/1
  q_B_I Integrator/1 -> q2dcm/1, q_B_I/1, Mux1/2
  Satellite Dynamic/1 -> Demux2/1
  Disturbances Torque/1 -> Add/1
  Demux2/2 -> " w_B_BI Integrator"/1
  Mux1/1 -> Satellite Dynamic/1
  Rotation Transformation/1 -> R_O_B Selector/1, R_B_I Selector/1, e_B_I Selector2/1, e_B_I Selector1/1, e_B_O Selector/1, R_O_I Selector/1
  " w_B_BI Integrator"/1 -> w_B_BI/1, Mux1/3
  Demux2/1 -> q_B_I Integrator/1
  Vector Concatenate/1 -> Rotation Transformation/1
  R_B_I Selector/1 -> R_B_I/1
  R_O_B Selector/1 -> R_O_B/1
  Control Torque/1 -> Add/2
  Add/1 -> Mux1/1
  e_B_I Selector1/1 -> e_B_I/1
  e_B_O Selector/1 -> e_B_O/1
  R_O_I_in/1 -> dcm2q1/1, Vector Concatenate/2
  q2dcm/1 -> Vector Concatenate/1
  e_B_I Selector2/1 -> dcm2q/1
  dcm2q/1 -> q_B_O/1
  dcm2q1/1 -> q_O_I/1

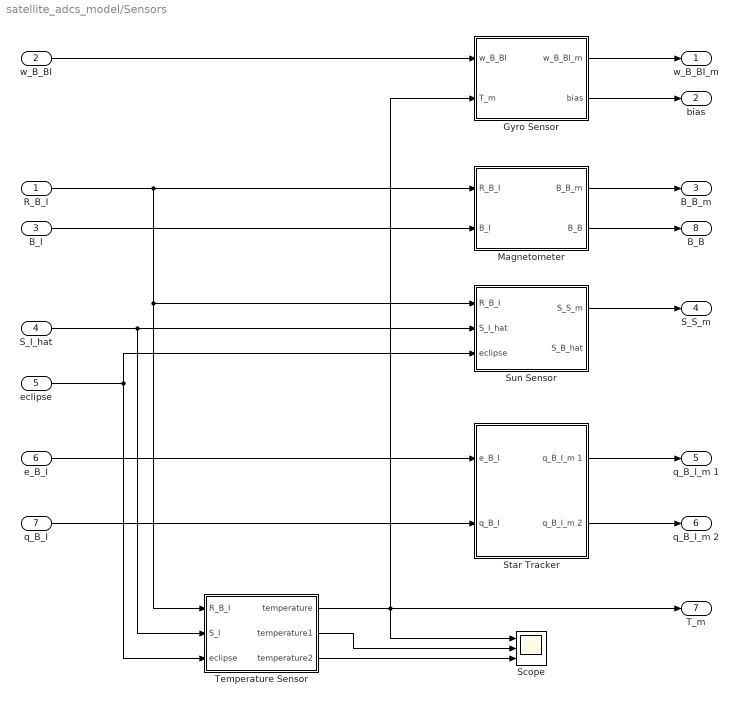
== system satellite_adcs_model/Sensors ==
  R_B_I : Inport
  w_B_BI : Inport  Port=2
  B_I : Inport  Port=3
  S_I_hat : Inport  Port=4
  eclipse : Inport  Port=5
  e_B_I : Inport  Port=6
  q_B_I : Inport  Port=7
  Gyro Sensor : Subsystem
  Magnetometer : Subsystem
  Scope : Scope  NumInputPorts=3
  Star Tracker : Subsystem
  Sun Sensor : Subsystem
  Temperature Sensor : Subsystem
  w_B_BI_m : Outport
  bias : Outport  Port=2
  B_B_m : Outport  Port=3
  S_S_m : Outport  Port=4
  q_B_I_m 1 : Outport  Port=5
  q_B_I_m 2 : Outport  Port=6
  T_m : Outport  Port=7
  B_B : Outport  Port=8
  wires:
  e_B_I/1 -> Star Tracker/1(e_B_I)
  B_I/1 -> Magnetometer/2(B_I)
  Sun Sensor/1(S_S_m) -> S_S_m/1
  Gyro Sensor/2(bias) -> bias/1
  Gyro Sensor/1(w_B_BI_m) -> w_B_BI_m/1
  Star Tracker/1(q_B_I_m 1) -> q_B_I_m 1/1
  Magnetometer/1(B_B_m) -> B_B_m/1
  w_B_BI/1 -> Gyro Sensor/1(w_B_BI)
  S_I_hat/1 -> Temperature Sensor/2(S_I), Sun Sensor/2(S_I_hat)
  R_B_I/1 -> Magnetometer/1(R_B_I), Temperature Sensor/1(R_B_I), Sun Sensor/1(R_B_I)
  q_B_I/1 -> Star Tracker/2(q_B_I)
  eclipse/1 -> Sun Sensor/3(eclipse), Temperature Sensor/3(eclipse)
  Star Tracker/2(q_B_I_m 2) -> q_B_I_m 2/1
  Temperature Sensor/2(temperature1) -> Scope/2
  Temperature Sensor/3(temperature2) -> Scope/3
  Temperature Sensor/1(temperature) -> Scope/1, T_m/1, Gyro Sensor/2(T_m)
  Magnetometer/2(B_B) -> B_B/1

== system satellite_adcs_model/Environmental Effect/DENSITY ==
  R : Inport
  S_TA : Inport  Port=2
  BETA : Inport  Port=3
  Environment Density : MATLABFcn  MATLABFcn=environmentDensity  OutputDimensions=1  Output1D=off
  Mux : Mux  Inputs=3
  RHO : Outport
  wires:
  Mux/1 -> Environment Density/1
  Environment Density/1 -> RHO/1
  BETA/1 -> Mux/3
  R/1 -> Mux/1
  S_TA/1 -> Mux/2

== system satellite_adcs_model/Environmental Effect/MAGNETIC FIELD ==
  R_I_E : Inport
  R : Inport  Port=2
  Derivative : Derivative
  Magnetic Field : MATLABFcn  MATLABFcn=environmentMagnetic  OutputDimensions=[3,1]  Output1D=off
  Vector Concatenate : Concatenate  Mode=Multidimensional array  ConcatenateDimension=2
  B_I : Outport
  Bdot_I : Outport  Port=2
  wires:
  Vector Concatenate/1 -> Magnetic Field/1
  R_I_E/1 -> Vector Concatenate/1
  R/1 -> Vector Concatenate/2
  Magnetic Field/1 -> Derivative/1, B_I/1
  Derivative/1 -> Bdot_I/1

== system satellite_adcs_model/Environmental Effect/SUN ==
  R : Inport
  S_TA : Inport  Port=2
  BETA : Inport  Port=3
  R_O_I : Inport  Port=4
  R_B_I : Inport  Port=5
  Mux1 : Mux  Inputs=3
  Selector : Selector  NumberOfDimensions=2  InputPortWidth=3  IndexOptions=Index vector (dialog),Index vector (dialog)  Indices=3,3  OutputSizes=1,1
  Selector1 : Selector  NumberOfDimensions=2  InputPortWidth=3  IndexOptions=Index vector (dialog),Index vector (dialog)  Indices=[1:3],1  OutputSizes=1,1
  Selector2 : Selector  NumberOfDimensions=2  InputPortWidth=3  IndexOptions=Index vector (dialog),Index vector (dialog)  Indices=[1:3],2  OutputSizes=1,1
  Sun Environment : MATLABFcn  MATLABFcn=environmentSun  OutputDimensions=[3,3]  Output1D=off
  Vector Concatenate1 : Concatenate  NumInputs=4  Mode=Multidimensional array  ConcatenateDimension=2
  S_B_hat : Outport
  S_I_hat : Outport  Port=2
  Eclipse : Outport  Port=3
  wires:
  Mux1/1 -> Vector Concatenate1/4
  R_B_I/1 -> Vector Concatenate1/3
  R_O_I/1 -> Vector Concatenate1/2
  Vector Concatenate1/1 -> Sun Environment/1
  Selector/1 -> Eclipse/1
  Selector1/1 -> S_B_hat/1
  Selector2/1 -> S_I_hat/1
  Sun Environment/1 -> Selector/1, Selector2/1, Selector1/1
  S_TA/1 -> Mux1/1
  BETA/1 -> Mux1/2
  R/1 -> Vector Concatenate1/1

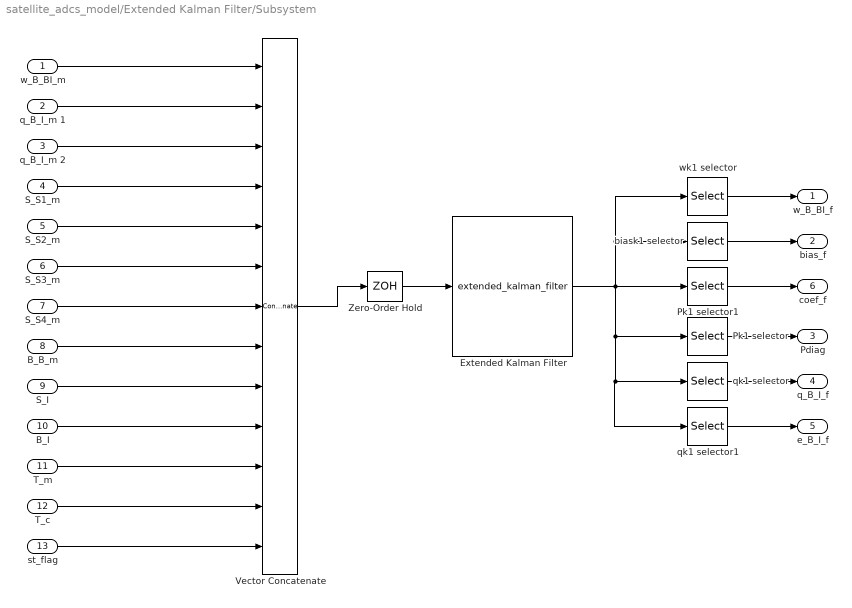
== system satellite_adcs_model/Extended Kalman Filter/Subsystem ==
  w_B_BI_m : Inport
  q_B_I_m 1 : Inport  Port=2
  q_B_I_m 2 : Inport  Port=3
  S_S1_m : Inport  Port=4
  S_S2_m : Inport  Port=5
  S_S3_m : Inport  Port=6
  S_S4_m : Inport  Port=7
  B_B_m : Inport  Port=8
  S_I : Inport  Port=9
  B_I : Inport  Port=10
  T_m : Inport  Port=11
  T_c : Inport  Port=12
  st_flag : Inport  Port=13
  Extended Kalman Filter : MATLABFcn  MATLABFcn=extended_kalman_filter  OutputDimensions=[12,14]  Output1D=off
  Pk1 selector : Selector  NumberOfDimensions=2  InputPortWidth=3  IndexOptions=Index vector (dialog),Index vector (dialog)  Indices=[1:12],[2:13]  OutputSizes=1,1
  Pk1 selector1 : Selector  NumberOfDimensions=2  InputPortWidth=3  IndexOptions=Index vector (dialog),Index vector (dialog)  Indices=[7:9],1  OutputSizes=1,1
  Vector Concatenate : Concatenate  NumInputs=13  Mode=Multidimensional array  ConcatenateDimension=2
  Zero-Order Hold : ZeroOrderHold  SampleTime=dt
  biask1 selector : Selector  NumberOfDimensions=2  InputPortWidth=3  IndexOptions=Index vector (dialog),Index vector (dialog)  Indices=[4:6],1  OutputSizes=1,1
  qk1 selector : Selector  NumberOfDimensions=2  InputPortWidth=3  IndexOptions=Index vector (dialog),Index vector (dialog)  Indices=[1:4],14  OutputSizes=1,1
  qk1 selector1 : Selector  NumberOfDimensions=2  InputPortWidth=3  IndexOptions=Index vector (dialog),Index vector (dialog)  Indices=[5:7],14  OutputSizes=1,1
  wk1 selector : Selector  NumberOfDimensions=2  InputPortWidth=3  IndexOptions=Index vector (dialog),Index vector (dialog)  Indices=[1:3],1  OutputSizes=1,1
  w_B_BI_f : Outport
  bias_f : Outport  Port=2
  Pdiag : Outport  Port=3
  q_B_I_f : Outport  Port=4
  e_B_I_f : Outport  Port=5
  coef_f : Outport  Port=6
  wires:
  Vector Concatenate/1 -> Zero-Order Hold/1
  S_S2_m/1 -> Vector Concatenate/5
  Pk1 selector/1 -> Pdiag/1
  qk1 selector1/1 -> e_B_I_f/1
  qk1 selector/1 -> q_B_I_f/1
  B_B_m/1 -> Vector Concatenate/8
  S_S1_m/1 -> Vector Concatenate/4
  S_I/1 -> Vector Concatenate/9
  q_B_I_m 1/1 -> Vector Concatenate/2
  wk1 selector/1 -> w_B_BI_f/1
  w_B_BI_m/1 -> Vector Concatenate/1
  B_I/1 -> Vector Concatenate/10
  biask1 selector/1 -> bias_f/1
  Zero-Order Hold/1 -> Extended Kalman Filter/1
  S_S3_m/1 -> Vector Concatenate/6
  S_S4_m/1 -> Vector Concatenate/7
  Pk1 selector1/1 -> coef_f/1
  Extended Kalman Filter/1 -> Pk1 selector1/1, qk1 selector1/1, qk1 selector/1, Pk1 selector/1, wk1 selector/1, biask1 selector/1
  T_m/1 -> Vector Concatenate/11
  q_B_I_m 2/1 -> Vector Concatenate/3
  T_c/1 -> Vector Concatenate/12
  st_flag/1 -> Vector Concatenate/13

== system satellite_adcs_model/Orbit Propagator/Sun Direction True Anomaly ==
  V : Inport
  R : Inport  Port=2
  S_I : Inport  Port=3
  Mux2 : Mux  Inputs=3
  sun_ta : MATLABFcn  MATLABFcn=sun_ta  OutputDimensions=[1,1]  Output1D=off
  ta : Outport
  wires:
  sun_ta/1 -> ta/1
  R/1 -> Mux2/1
  V/1 -> Mux2/2
  S_I/1 -> Mux2/3
  Mux2/1 -> sun_ta/1

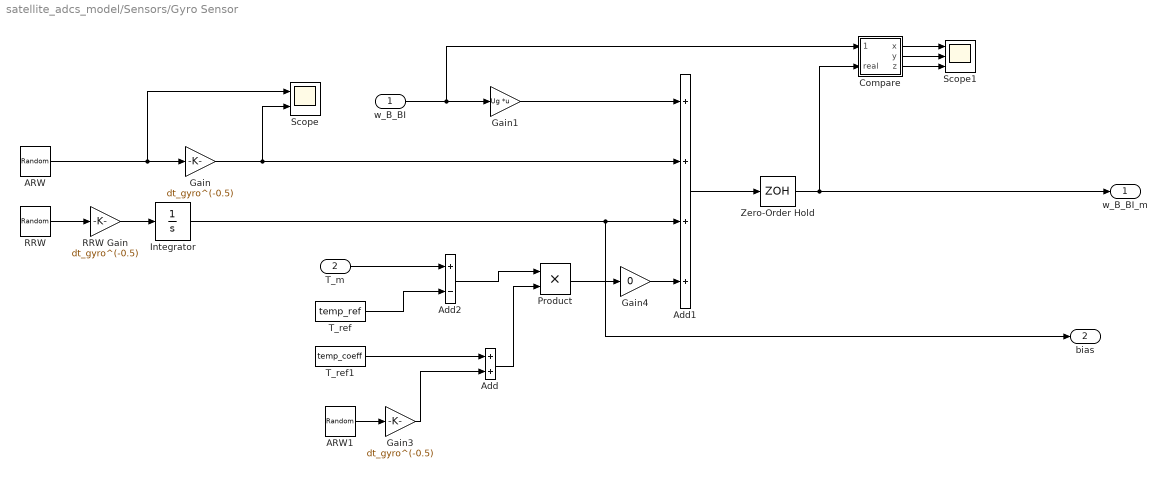
== system satellite_adcs_model/Sensors/Gyro Sensor ==
  w_B_BI : Inport
  T_m : Inport  Port=2
  ARW : RandomNumber  Variance=[Var_ARW;Var_ARW;Var_ARW]  SampleTime=dt  VectorParams1D=off
  ARW1 : RandomNumber  Variance=[VarW;VarW;VarW]  SampleTime=dt  VectorParams1D=off
  Add : Sum
  Add1 : Sum  Inputs=++++
  Add2 : Sum  Inputs=+-
  Compare : Subsystem
  Gain : Gain  Gain=dt_gyro^(-0.5)
  Gain1 : Gain  Gain=Ug  Multiplication=Matrix(K*u)
  Gain3 : Gain  Gain=dt_gyro^(-0.5)
  Gain4 : Gain  Gain=0
  Integrator : Integrator  InitialCondition=GYRO_Bias
  Product : Product
  RRW : RandomNumber  Variance=[Var_RRW;Var_RRW;Var_RRW]  SampleTime=dt  VectorParams1D=off
  RRW Gain : Gain  Gain=dt_gyro^(-0.5)
  Scope : Scope  NumInputPorts=2
  Scope1 : Scope  NumInputPorts=3
  T_ref : Constant  Value=temp_ref
  T_ref1 : Constant  Value=temp_coeff  VectorParams1D=off
  Zero-Order Hold : ZeroOrderHold  SampleTime=dt
  w_B_BI_m : Outport
  bias : Outport  Port=2
  wires:
  w_B_BI/1 -> Gain1/1, Compare/1(true)
  Gain/1 -> Scope/2, Add1/2
  ARW/1 -> Scope/1, Gain/1
  Add1/1 -> Zero-Order Hold/1
  Gain1/1 -> Add1/1
  Zero-Order Hold/1 -> w_B_BI_m/1, Compare/2(real)
  Compare/2(y) -> Scope1/2
  Compare/3(z) -> Scope1/3
  Compare/1(x) -> Scope1/1
  RRW/1 -> RRW Gain/1
  Integrator/1 -> Add1/3, bias/1
  RRW Gain/1 -> Integrator/1
  Add2/1 -> Product/1
  T_m/1 -> Add2/1
  Product/1 -> Gain4/1
  T_ref/1 -> Add2/2
  Add/1 -> Product/2
  T_ref1/1 -> Add/1
  ARW1/1 -> Gain3/1
  Gain3/1 -> Add/2
  Gain4/1 -> Add1/4

== system satellite_adcs_model/Sensors/Magnetometer ==
  R_B_I : Inport
  B_I : Inport  Port=2
  ARW : RandomNumber  Variance=[sigMag^2;sigMag^2;sigMag^2]  SampleTime=dt_mg  VectorParams1D=off
  Add1 : Sum
  Compare : Subsystem
  Matrix Multiply : Product  Multiplication=Matrix(*)
  ScaleFactor MissAlignment : Gain  Gain=Umg  Multiplication=Matrix(K*u)
  Scope1 : Scope  NumInputPorts=3
  Zero-Order Hold : ZeroOrderHold  SampleTime=dt_mg
  B_B_m : Outport
  B_B : Outport  Port=2
  wires:
  Matrix Multiply/1 -> B_B/1, Compare/1(true), ScaleFactor MissAlignment/1  "B_B"
  ScaleFactor MissAlignment/1 -> Add1/1
  Add1/1 -> Zero-Order Hold/1
  ARW/1 -> Add1/2
  B_I/1 -> Matrix Multiply/2
  R_B_I/1 -> Matrix Multiply/1
  Compare/2(y) -> Scope1/2
  Compare/3(z) -> Scope1/3
  Compare/1(x) -> Scope1/1
  Zero-Order Hold/1 -> Compare/2(real), B_B_m/1

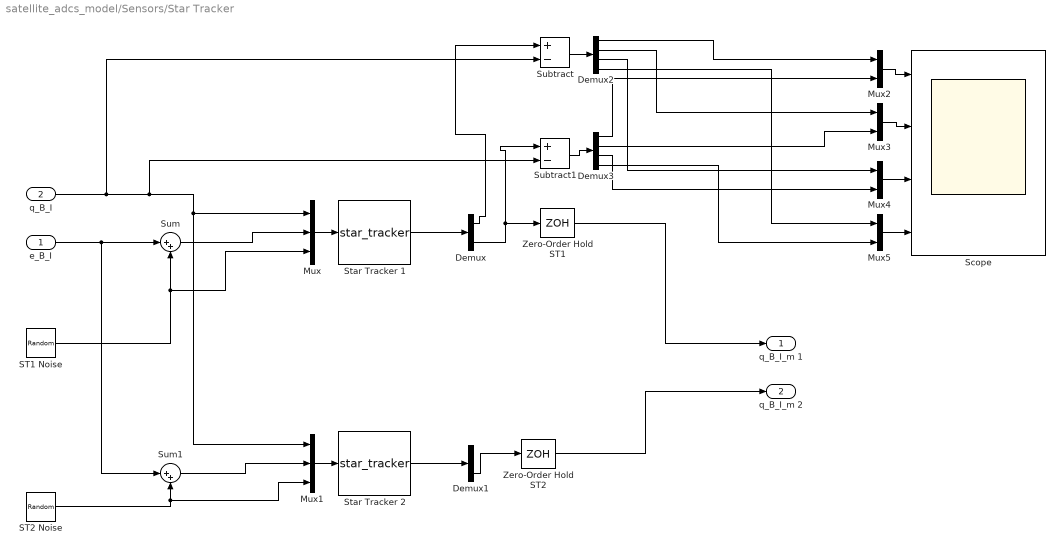
== system satellite_adcs_model/Sensors/Star Tracker ==
  e_B_I : Inport
  q_B_I : Inport  Port=2
  Demux : Demux  Outputs=2
  Demux1 : Demux  Outputs=2
  Demux2 : Demux
  Demux3 : Demux
  Mux : Mux  Inputs=3
  Mux1 : Mux  Inputs=3
  Mux{2..5} (4 alike) : Mux  Inputs=2
  ST1 Noise : RandomNumber  Variance=[varST_x(1);varST_y(1);varST_z(1)]  SampleTime=dt  VectorParams1D=off
  ST2 Noise : RandomNumber  Variance=[varST_x(2);varST_y(2);varST_z(2)]  SampleTime=dt  VectorParams1D=off
  Scope : Scope  NumInputPorts=4
  Star Tracker 1 : MATLABFcn  MATLABFcn=star_tracker  OutputDimensions=[8,1]  Output1D=off
  Star Tracker 2 : MATLABFcn  MATLABFcn=star_tracker  OutputDimensions=[8,1]  Output1D=off
  Subtract : Sum  Inputs=+-
  Subtract1 : Sum  Inputs=+-
  Sum : Sum  Inputs=|++
  Sum1 : Sum  Inputs=|++
  Zero-Order Hold ST1 : ZeroOrderHold  SampleTime=dt_st
  Zero-Order Hold ST2 : ZeroOrderHold  SampleTime=dt_st
  q_B_I_m 1 : Outport
  q_B_I_m 2 : Outport  Port=2
  wires:
  Mux/1 -> Star Tracker 1/1
  q_B_I/1 -> Subtract/2, Subtract1/2, Mux1/1, Mux/1
  ST1 Noise/1 -> Mux/3, Sum/2
  Sum/1 -> Mux/2
  Sum1/1 -> Mux1/2
  e_B_I/1 -> Sum1/1, Sum/1
  Star Tracker 2/1 -> Demux1/1
  ST2 Noise/1 -> Mux1/3, Sum1/2
  Mux1/1 -> Star Tracker 2/1
  Zero-Order Hold ST1/1 -> q_B_I_m 1/1
  Zero-Order Hold ST2/1 -> q_B_I_m 2/1
  Star Tracker 1/1 -> Demux/1
  Demux/1 -> Subtract/1
  Demux1/2 -> Zero-Order Hold ST2/1
  Demux2/1 -> Mux2/1
  Demux/2 -> Zero-Order Hold ST1/1, Subtract1/1
  Subtract/1 -> Demux2/1
  Subtract1/1 -> Demux3/1
  Mux2/1 -> Scope/1
  Mux3/1 -> Scope/2
  Mux4/1 -> Scope/3
  Mux5/1 -> Scope/4
  Demux2/2 -> Mux3/1
  Demux2/3 -> Mux4/1
  Demux2/4 -> Mux5/1
  Demux3/1 -> Mux2/2
  Demux3/2 -> Mux3/2
  Demux3/3 -> Mux4/2
  Demux3/4 -> Mux5/2

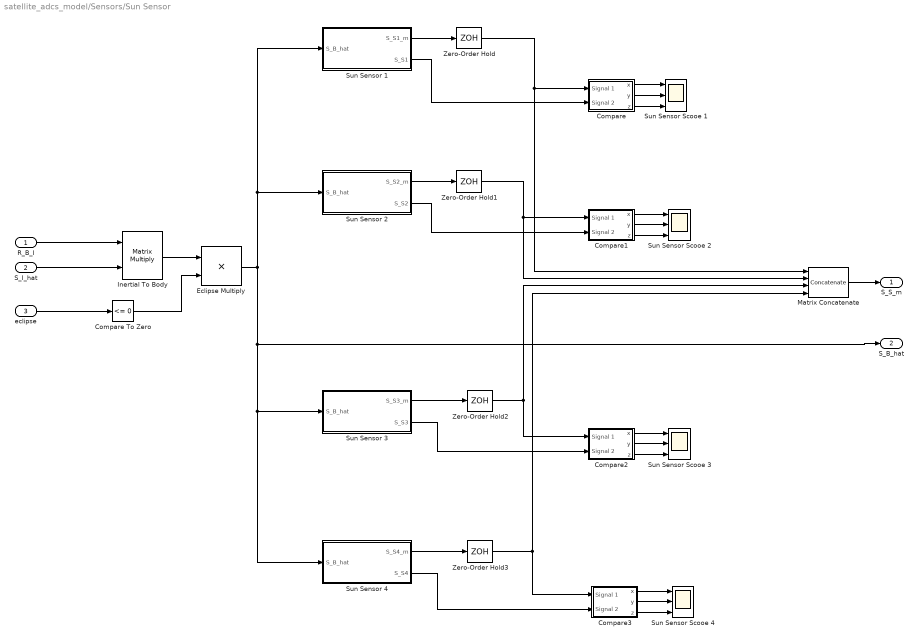
== system satellite_adcs_model/Sensors/Sun Sensor ==
  R_B_I : Inport
  S_I_hat : Inport  Port=2
  eclipse : Inport  Port=3
  Compare : Subsystem
  Compare To Zero : simulink/Logic and Bit Operations/Compare To Zero  relop=<=  OutDataTypeStr=boolean
  Compare1 : Subsystem
  Compare2 : Subsystem
  Compare3 : Subsystem
  Eclipse Multiply : Product
  Inertial To Body : Product  Multiplication=Matrix(*)
  Matrix Concatenate : Concatenate  NumInputs=4  Mode=Multidimensional array  ConcatenateDimension=2
  Sun Sensor Scooe {1..4} (4 alike) : Scope  NumInputPorts=3
  Sun Sensor 1 : Subsystem
  Sun Sensor 2 : Subsystem
  Sun Sensor 3 : Subsystem
  Sun Sensor 4 : Subsystem
  Zero-Order Hold{,1..3} (4 alike) : ZeroOrderHold  SampleTime=dt_ss
  S_S_m : Outport
  S_B_hat : Outport  Port=2
  wires:
  R_B_I/1 -> Inertial To Body/1
  Eclipse Multiply/1 -> Sun Sensor 1/1(S_B_hat), Sun Sensor 2/1(S_B_hat), Sun Sensor 4/1(S_B_hat), Sun Sensor 3/1(S_B_hat), S_B_hat/1
  Matrix Concatenate/1 -> S_S_m/1
  Inertial To Body/1 -> Eclipse Multiply/1
  Compare To Zero/1 -> Eclipse Multiply/2
  eclipse/1 -> Compare To Zero/1
  Sun Sensor 1/1(S_S1_m) -> Zero-Order Hold/1
  Sun Sensor 2/1(S_S2_m) -> Zero-Order Hold1/1
  Zero-Order Hold/1 -> Compare/1(Signal 1), Matrix Concatenate/1
  Zero-Order Hold1/1 -> Compare1/1(Signal 1), Matrix Concatenate/2
  Sun Sensor 1/2(S_S1) -> Compare/2(Signal 2)
  Compare/1(x) -> Sun Sensor Scooe 1/1
  Compare/2(y) -> Sun Sensor Scooe 1/2
  Compare/3(z) -> Sun Sensor Scooe 1/3
  Sun Sensor 3/1(S_S3_m) -> Zero-Order Hold2/1
  Sun Sensor 4/1(S_S4_m) -> Zero-Order Hold3/1
  Zero-Order Hold2/1 -> Compare2/1(Signal 1), Matrix Concatenate/3
  Zero-Order Hold3/1 -> Compare3/1(Signal 1), Matrix Concatenate/4
  Compare1/2(y) -> Sun Sensor Scooe 2/2
  Compare1/1(x) -> Sun Sensor Scooe 2/1
  Compare1/3(z) -> Sun Sensor Scooe 2/3
  Sun Sensor 2/2(S_S2) -> Compare1/2(Signal 2)
  Compare2/2(y) -> Sun Sensor Scooe 3/2
  Compare2/1(x) -> Sun Sensor Scooe 3/1
  Compare2/3(z) -> Sun Sensor Scooe 3/3
  Sun Sensor 3/2(S_S3) -> Compare2/2(Signal 2)
  Compare3/2(y) -> Sun Sensor Scooe 4/2
  Compare3/1(x) -> Sun Sensor Scooe 4/1
  Compare3/3(z) -> Sun Sensor Scooe 4/3
  Sun Sensor 4/2(S_S4) -> Compare3/2(Signal 2)
  S_I_hat/1 -> Inertial To Body/2

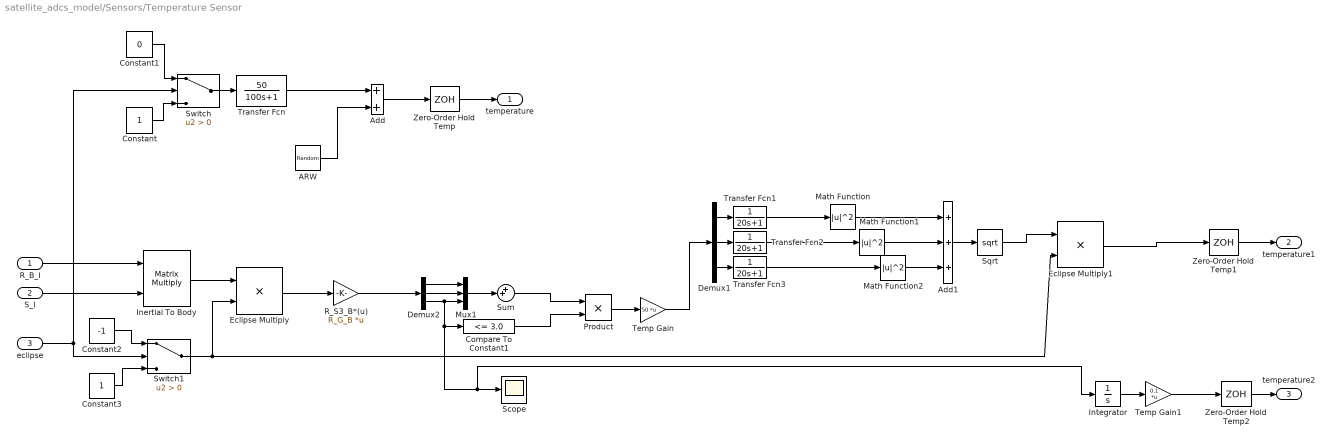
== system satellite_adcs_model/Sensors/Temperature Sensor ==
  R_B_I : Inport
  S_I : Inport  Port=2
  eclipse : Inport  Port=3
  ARW : RandomNumber  Variance=varTemp  SampleTime=dt  VectorParams1D=off
  Add : Sum
  Add1 : Sum  Inputs=+++
  Compare To Constant1 : simulink/Logic and Bit Operations/Compare To Constant  relop=<=  const=3.0  OutDataTypeStr=boolean
  Constant : Constant
  Constant1 : Constant  Value=0
  Constant2 : Constant  Value=-1
  Constant3 : Constant
  Demux1 : Demux  Outputs=3
  Demux2 : Demux  Outputs=3
  Eclipse Multiply : Product
  Eclipse Multiply1 : Product
  Inertial To Body : Product  Multiplication=Matrix(*)
  Integrator : Integrator
  Math Function : Math  Operator=magnitude^2  SaturateOnIntegerOverflow=on
  Math Function1 : Math  Operator=magnitude^2  SaturateOnIntegerOverflow=on
  Math Function2 : Math  Operator=magnitude^2  SaturateOnIntegerOverflow=on
  Mux1 : Mux  Inputs=3
  Product : Product
  R_S3_B*(u) : Gain  Gain=R_G_B  Multiplication=Matrix(K*u)
  Scope : Scope
  Sqrt : Sqrt  SaturateOnIntegerOverflow=on
  Sum : Sum  Inputs=++|
  Switch : Switch  Criteria=u2 > Threshold
  Switch1 : Switch  Criteria=u2 > Threshold
  Temp Gain : Gain  Gain=50  Multiplication=Matrix(K*u)
  Temp Gain1 : Gain  Gain=0.1  Multiplication=Matrix(K*u)
  Transfer Fcn : TransferFcn  Numerator=[50]  Denominator=[100 1]
  Transfer Fcn1 : TransferFcn  Numerator=1  Denominator=[20 1]
  Transfer Fcn2 : TransferFcn  Denominator=[20 1]
  Transfer Fcn3 : TransferFcn  Denominator=[20 1]
  Zero-Order Hold Temp : ZeroOrderHold  SampleTime=dt_ts
  Zero-Order Hold Temp1 : ZeroOrderHold  SampleTime=dt_ts
  Zero-Order Hold Temp2 : ZeroOrderHold  SampleTime=dt_ts
  temperature : Outport
  temperature1 : Outport  Port=2
  temperature2 : Outport  Port=3
  wires:
  Transfer Fcn/1 -> Add/1
  Switch/1 -> Transfer Fcn/1
  Constant/1 -> Switch/3
  Constant1/1 -> Switch/1
  Add/1 -> Zero-Order Hold Temp/1
  ARW/1 -> Add/2
  Zero-Order Hold Temp/1 -> temperature/1
  S_I/1 -> Inertial To Body/2
  Inertial To Body/1 -> Eclipse Multiply/1
  R_B_I/1 -> Inertial To Body/1
  eclipse/1 -> Switch1/2, Switch/2
  Demux2/1 -> Mux1/1
  Demux2/2 -> Mux1/2
  R_S3_B*(u)/1 -> Demux2/1
  Eclipse Multiply/1 -> R_S3_B*(u)/1
  Mux1/1 -> Sum/2
  Demux2/3 -> Integrator/1, Scope/1, Compare To Constant1/1, Mux1/3
  Sum/1 -> Product/1
  Compare To Constant1/1 -> Product/2
  Zero-Order Hold Temp1/1 -> temperature1/1
  Product/1 -> Temp Gain/1
  Temp Gain/1 -> Demux1/1
  Transfer Fcn3/1 -> Math Function2/1
  Demux1/1 -> Transfer Fcn1/1
  Demux1/2 -> Transfer Fcn2/1
  Transfer Fcn1/1 -> Math Function/1
  Transfer Fcn2/1 -> Math Function1/1
  Zero-Order Hold Temp2/1 -> temperature2/1
  Demux1/3 -> Transfer Fcn3/1
  Add1/1 -> Sqrt/1
  Math Function1/1 -> Add1/2
  Math Function2/1 -> Add1/3
  Math Function/1 -> Add1/1
  Sqrt/1 -> Eclipse Multiply1/1
  Constant3/1 -> Switch1/3
  Constant2/1 -> Switch1/1
  Switch1/1 -> Eclipse Multiply1/2, Eclipse Multiply/2
  Eclipse Multiply1/1 -> Zero-Order Hold Temp1/1
  Integrator/1 -> Temp Gain1/1
  Temp Gain1/1 -> Zero-Order Hold Temp2/1

== system satellite_adcs_model/Sensors/Gyro Sensor/Compare ==
  true : Inport
  real : Inport  Port=2
  Demux : Demux  Outputs=3
  Demux1 : Demux  Outputs=3
  Mux : Mux  Inputs=2
  Mux1 : Mux  Inputs=2
  Mux2 : Mux  Inputs=2
  x : Outport
  y : Outport  Port=2
  z : Outport  Port=3
  wires:
  Mux1/1 -> y/1
  Mux2/1 -> z/1
  true/1 -> Demux/1
  real/1 -> Demux1/1
  Mux/1 -> x/1
  Demux1/3 -> Mux2/2
  Demux1/2 -> Mux1/2
  Demux/3 -> Mux2/1
  Demux/1 -> Mux/1
  Demux/2 -> Mux1/1
  Demux1/1 -> Mux/2

== system satellite_adcs_model/Sensors/Magnetometer/Compare ==
  true : Inport
  real : Inport  Port=2
  Demux : Demux  Outputs=3
  Demux1 : Demux  Outputs=3
  Mux : Mux  Inputs=2
  Mux1 : Mux  Inputs=2
  Mux2 : Mux  Inputs=2
  x : Outport
  y : Outport  Port=2
  z : Outport  Port=3
  wires:
  Mux1/1 -> y/1
  Mux2/1 -> z/1
  true/1 -> Demux/1
  real/1 -> Demux1/1
  Mux/1 -> x/1
  Demux1/3 -> Mux2/2
  Demux1/2 -> Mux1/2
  Demux/3 -> Mux2/1
  Demux/1 -> Mux/1
  Demux/2 -> Mux1/1
  Demux1/1 -> Mux/2

== system satellite_adcs_model/Sensors/Sun Sensor/Compare ==
  Signal 1 : Inport
  Signal 2 : Inport  Port=2
  Demux3 : Demux  Outputs=3
  Demux4 : Demux  Outputs=3
  Mux : Mux  Inputs=2
  Mux1 : Mux  Inputs=2
  Mux2 : Mux  Inputs=2
  x : Outport
  y : Outport  Port=2
  z : Outport  Port=3
  wires:
  Demux3/3 -> Mux2/2
  Demux3/2 -> Mux1/2
  Demux4/2 -> Mux1/1
  Demux3/1 -> Mux/2
  Mux/1 -> x/1
  Mux2/1 -> z/1
  Demux4/1 -> Mux/1
  Mux1/1 -> y/1
  Demux4/3 -> Mux2/1
  Signal 2/1 -> Demux3/1
  Signal 1/1 -> Demux4/1

== system satellite_adcs_model/Sensors/Sun Sensor/Compare1 ==
  Signal 1 : Inport
  Signal 2 : Inport  Port=2
  Demux3 : Demux  Outputs=3
  Demux4 : Demux  Outputs=3
  Mux : Mux  Inputs=2
  Mux1 : Mux  Inputs=2
  Mux2 : Mux  Inputs=2
  x : Outport
  y : Outport  Port=2
  z : Outport  Port=3
  wires:
  Demux3/3 -> Mux2/2
  Demux3/2 -> Mux1/2
  Demux4/2 -> Mux1/1
  Demux3/1 -> Mux/2
  Mux/1 -> x/1
  Mux2/1 -> z/1
  Demux4/1 -> Mux/1
  Mux1/1 -> y/1
  Demux4/3 -> Mux2/1
  Signal 2/1 -> Demux3/1
  Signal 1/1 -> Demux4/1

== system satellite_adcs_model/Sensors/Sun Sensor/Compare2 ==
  Signal 1 : Inport
  Signal 2 : Inport  Port=2
  Demux3 : Demux  Outputs=3
  Demux4 : Demux  Outputs=3
  Mux : Mux  Inputs=2
  Mux1 : Mux  Inputs=2
  Mux2 : Mux  Inputs=2
  x : Outport
  y : Outport  Port=2
  z : Outport  Port=3
  wires:
  Demux3/3 -> Mux2/2
  Demux3/2 -> Mux1/2
  Demux4/2 -> Mux1/1
  Demux3/1 -> Mux/2
  Mux/1 -> x/1
  Mux2/1 -> z/1
  Demux4/1 -> Mux/1
  Mux1/1 -> y/1
  Demux4/3 -> Mux2/1
  Signal 2/1 -> Demux3/1
  Signal 1/1 -> Demux4/1

== system satellite_adcs_model/Sensors/Sun Sensor/Compare3 ==
  Signal 1 : Inport
  Signal 2 : Inport  Port=2
  Demux3 : Demux  Outputs=3
  Demux4 : Demux  Outputs=3
  Mux : Mux  Inputs=2
  Mux1 : Mux  Inputs=2
  Mux2 : Mux  Inputs=2
  x : Outport
  y : Outport  Port=2
  z : Outport  Port=3
  wires:
  Demux3/3 -> Mux2/2
  Demux3/2 -> Mux1/2
  Demux4/2 -> Mux1/1
  Demux3/1 -> Mux/2
  Mux/1 -> x/1
  Mux2/1 -> z/1
  Demux4/1 -> Mux/1
  Mux1/1 -> y/1
  Demux4/3 -> Mux2/1
  Signal 2/1 -> Demux3/1
  Signal 1/1 -> Demux4/1

== system satellite_adcs_model/Sensors/Sun Sensor/Sun Sensor 1 ==
  S_B_hat : Inport
  Compare To Constant : simulink/Logic and Bit Operations/Compare To Constant  relop=<=  const=3.0  OutDataTypeStr=boolean
  Demux1 : Demux  Outputs=3
  Mux : Mux  Inputs=3
  Product1 : Product
  R_S1_B : Gain  Gain=R_S1_B  Multiplication=Matrix(K*u)
  SS Noise : RandomNumber  Variance=(sigSS*pi/180)^2  SampleTime=dt_ss
  Sum : Sum  Inputs=++|
  S_S1_m : Outport
  S_S1 : Outport  Port=2
  wires:
  S_B_hat/1 -> R_S1_B/1
  Demux1/2 -> Mux/2
  Demux1/3 -> Compare To Constant/1, Mux/3
  Demux1/1 -> Mux/1
  Compare To Constant/1 -> Product1/2
  Product1/1 -> S_S1_m/1
  Sum/1 -> Product1/1
  Mux/1 -> Sum/2
  SS Noise/1 -> Sum/1
  R_S1_B/1 -> S_S1/1, Demux1/1

== system satellite_adcs_model/Sensors/Sun Sensor/Sun Sensor 2 ==
  S_B_hat : Inport
  Compare To Constant1 : simulink/Logic and Bit Operations/Compare To Constant  relop=<=  const=3.0  OutDataTypeStr=boolean
  Demux2 : Demux  Outputs=3
  Mux1 : Mux  Inputs=3
  Product : Product
  R_S2_B : Gain  Gain=R_S2_B  Multiplication=Matrix(K*u)
  SS Noise : RandomNumber  Variance=(sigSS*pi/180)^2  SampleTime=dt_ss
  Sum : Sum  Inputs=++|
  S_S2_m : Outport
  S_S2 : Outport  Port=2
  wires:
  Product/1 -> S_S2_m/1
  R_S2_B/1 -> S_S2/1, Demux2/1
  Demux2/1 -> Mux1/1
  Demux2/2 -> Mux1/2
  Demux2/3 -> Compare To Constant1/1, Mux1/3
  Compare To Constant1/1 -> Product/2
  S_B_hat/1 -> R_S2_B/1
  Sum/1 -> Product/1
  SS Noise/1 -> Sum/1
  Mux1/1 -> Sum/2

== system satellite_adcs_model/Sensors/Sun Sensor/Sun Sensor 3 ==
  S_B_hat : Inport
  Compare To Constant1 : simulink/Logic and Bit Operations/Compare To Constant  relop=<=  const=3.0  OutDataTypeStr=boolean
  Demux2 : Demux  Outputs=3
  Mux1 : Mux  Inputs=3
  Product : Product
  R_S3_B : Gain  Gain=R_S3_B  Multiplication=Matrix(K*u)
  SS Noise : RandomNumber  Variance=(sigSS*pi/180)^2  SampleTime=dt_ss
  Sum : Sum  Inputs=++|
  S_S3_m : Outport
  S_S3 : Outport  Port=2
  wires:
  Product/1 -> S_S3_m/1
  R_S3_B/1 -> S_S3/1, Demux2/1
  Demux2/1 -> Mux1/1
  Demux2/2 -> Mux1/2
  Demux2/3 -> Compare To Constant1/1, Mux1/3
  Compare To Constant1/1 -> Product/2
  S_B_hat/1 -> R_S3_B/1
  Sum/1 -> Product/1
  SS Noise/1 -> Sum/1
  Mux1/1 -> Sum/2
